simulink model "truck_fra_oven_konstant_hastighet"  (R2023b)
settings: Solver=VariableStepAuto  StartTime=0.0  StopTime=30  MaxStep=0.01  RelTol=1e-3
values from neighbouring files (symbols this model uses):
  k_1 = -0.1    [truck_fra_oven_konstant_hastighet_script.m]
  k_2 = 2    [truck_fra_oven_konstant_hastighet_script.m]
  y_r = 2    [truck_fra_oven_konstant_hastighet_script.m]
settings Model: Creator=hansae  LastModifiedBy=fredr
settings SolverCC: AlgebraicLoopSolver=TrustRegion
settings SFSimCC: CustomCodeUndefinedFunction=UseInterfaceOnly

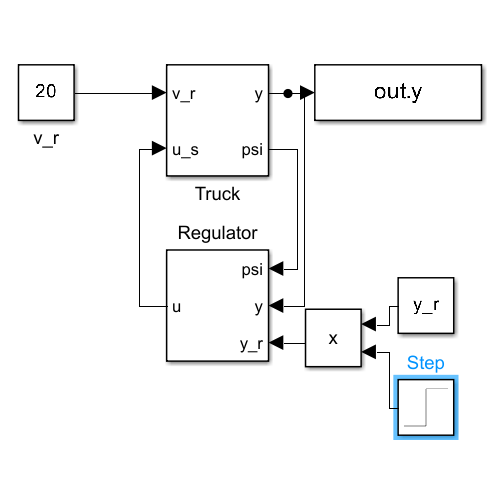
[thumbnail: Simulink's stored preview of the top-level diagram]
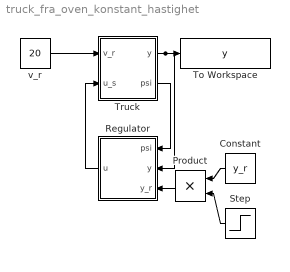
== system truck_fra_oven_konstant_hastighet ==
  Constant : Constant  Value=y_r
  Product : Product
  Regulator : Subsystem
  Step : Step  Time=10  Before=-1  SampleTime=0
  To Workspace : ToWorkspace  VariableName=y  SampleTime=-1
  Truck : Subsystem
  v_r : Constant  Value=20
  wires:
  v_r/1 -> Truck/1(v_r)
  Regulator/1(u) -> Truck/2(u_s)
  Truck/2(psi) -> Regulator/1(psi)
  Truck/1(y) -> To Workspace/1, Regulator/2(y)
  Product/1 -> Regulator/3(y_r)
  Constant/1 -> Product/1
  Step/1 -> Product/2

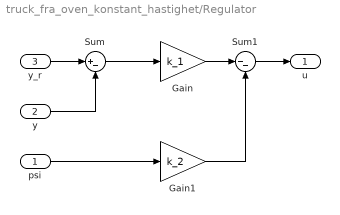
== system truck_fra_oven_konstant_hastighet/Regulator ==
  psi : Inport
  y : Inport  Port=2
  y_r : Inport  Port=3
  Gain : Gain  Gain=k_1
  Gain1 : Gain  Gain=k_2
  Sum : Sum  Inputs=|+-
  Sum1 : Sum  Inputs=|--
  u : Outport
  wires:
  y_r/1 -> Sum/1
  y/1 -> Sum/2
  Sum/1 -> Gain/1
  psi/1 -> Gain1/1
  Gain/1 -> Sum1/1
  Sum1/1 -> u/1
  Gain1/1 -> Sum1/2

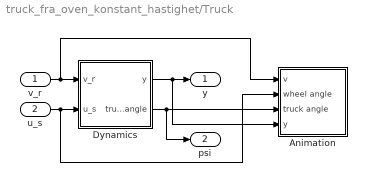
== system truck_fra_oven_konstant_hastighet/Truck ==
  v_r : Inport
  u_s : Inport  Port=2
  Animation : Subsystem
  Dynamics : Subsystem  ClipboardFcn=parameters_truck.m
  y : Outport
  psi : Outport  Port=2
  wires:
  Dynamics/1(y) -> Animation/4(y), y/1
  u_s/1 -> Animation/2(wheel angle), Dynamics/2(u_s)
  v_r/1 -> Animation/1(v), Dynamics/1(v_r)
  Dynamics/2(truck angle) -> psi/1, Animation/3(truck angle)

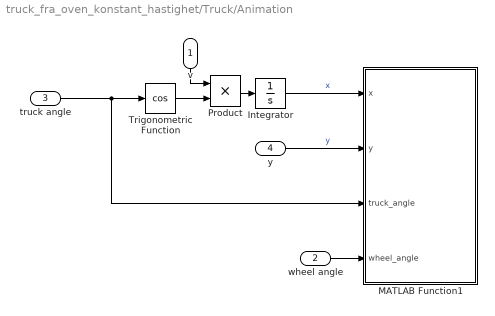
== system truck_fra_oven_konstant_hastighet/Truck/Animation ==
  v : Inport
  wheel angle : Inport  Port=2
  truck angle : Inport  Port=3
  y : Inport  Port=4
  Integrator : Integrator
  MATLAB Function1 : MATLAB Function  TreatAsAtomicUnit=on  SystemSampleTime=1/30
  Product : Product
  Trigonometric Function : Trigonometry  Operator=cos
  wires:
  Product/1 -> Integrator/1
  Trigonometric Function/1 -> Product/2
  v/1 -> Product/1
  y/1 -> MATLAB Function1/2(y)  "y"
  Integrator/1 -> MATLAB Function1/1(x)  "x"
  truck angle/1 -> MATLAB Function1/3(truck_angle), Trigonometric Function/1
  wheel angle/1 -> MATLAB Function1/4(wheel_angle)

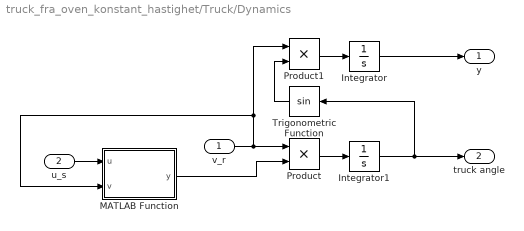
== system truck_fra_oven_konstant_hastighet/Truck/Dynamics ==
  v_r : Inport
  u_s : Inport  Port=2
  Integrator : Integrator  InitialCondition=-2
  Integrator1 : Integrator
  MATLAB Function : MATLAB Function  TreatAsAtomicUnit=on
  Product : Product
  Product1 : Product
  Trigonometric Function : Trigonometry
  y : Outport
  truck angle : Outport  Port=2
  wires:
  Integrator/1 -> y/1
  Integrator1/1 -> truck angle/1, Trigonometric Function/1
  Product/1 -> Integrator1/1
  v_r/1 -> MATLAB Function/2(v), Product1/1, Product/1
  Product1/1 -> Integrator/1
  Trigonometric Function/1 -> Product1/2
  u_s/1 -> MATLAB Function/1(u)
  MATLAB Function/1(y) -> Product/2

== matlab function truck_fra_oven_konstant_hastighet/Truck/Dynamics/MATLAB Function ==
  data: u input; y output; v input
function y = saturation(u,v)
    Pmax = 400000;
    epsilon = 0.1;
    
    sat = Pmax/sqrt(v^2+epsilon);
    y = max(min(u,sat),-sat);

== matlab function truck_fra_oven_konstant_hastighet/Truck/Animation/MATLAB Function1 ==
  settings: updateMethod=DISCRETE
  data: x input; y input; truck_angle input; wheel_angle input
function plot_truck(x,y,truck_angle,wheel_angle)
    % Parameters
    l = 8;
    persistent Truck;

    % Plotting Truck
    if isempty(Truck)
        Truck = initialize_plot();
    else
        update_truck_position(Truck,x,y,truck_angle,wheel_angle);
    end    

    drawnow;

    % Functions
    function Truck = initialize_plot()
        % Create figure
        figure('position',[100,100,1500,500]);
        clf; grid on; hold on; daspect([1,1,1]);
        xlim([-20, 50])
        ylim([-10, 10])
    
        % Road
        plot([-5000,5000],[-4,-4],'k','linewidth',3);
        plot([-5000,5000],[4,4],'k','linewidth',3);
        plot([-5000,5000],[0,0],'y','linewidth',3);

        % Truck
        Truck               = hgtransform('parent',gca);
        Left_front_wheel    = hgtransform('parent',Truck);
        Right_front_wheel   = hgtransform('parent',Truck);

        % Back wheels
        rectangle('Position',[l/6,-l/100,l/8,l/40],'parent',Truck,'edgecolor','k','linewidth',2,'FaceColor','w')
        rectangle('Position',[l/6,l-2*l/3-(l/40-l/100),l/8,l/40],'parent',Truck,'edgecolor','k','linewidth',2,'FaceColor','w')
        % Front wheel
        rectangle('Position',[2*l/3+l/20,-l/100,l/8,l/40],'parent',Right_front_wheel,'edgecolor','k','linewidth',2,'FaceColor','w')
        rectangle('Position',[2*l/3+l/20,l-2*l/3-(l/40-l/100),l/8,l/40],'parent',Left_front_wheel,'edgecolor','k','linewidth',2,'FaceColor','w')
        % Back
        rectangle('Position',[0,0,11*l/18,l-2*l/3],'parent',Truck,'edgecolor','k','linewidth',2,'FaceColor','w')
        % Front
        rectangle('Position',[2*l/3,0,l-2*l/3,l-2*l/3],'parent',Truck,'edgecolor','k','linewidth',2,'FaceColor','w')
        % Connection
        rectangle('Position',[11*l/18,3*l/8-l/3,2*l/3-11*l/18,l-3*l/4],'parent',Truck,'edgecolor','k','linewidth',2,'FaceColor','w')
        % Window
        rectangle('Position',[7*l/8,0,l/8,l-2*l/3],'parent',Truck,'edgecolor','k','linewidth',2,'FaceColor','w')
        
    end
    
    function update_truck_position(Truck,x,y,truck_angle,wheel_angle)
        if ishandle(Truck)
            set(Truck, 'Matrix', makehgtform('translate', [x, y, 0], 'zrotate', truck_angle, 'translate', [-l/6-l/16, -l/2+l/3, 0]));
            
            children = get(Truck, 'Children');
            set(children(8), 'Matrix', makehgtform('translate', -[-(2*l/3+l/20)-l/16, -(l-2*l/3-(l/40-l/100))-l/80, 0], 'zrotate', -wheel_angle, 'translate', [-(2*l/3+l/20)-l/16, -(l-2*l/3-(l/40-l/100))-l/80, 0]));
            set(children(7), 'Matrix', makehgtform('translate', -[-(2*l/3+l/20)-l/16, l/100-l/80, 0], 'zrotate', -wheel_angle, 'translate', [-(2*l/3+l/20)-l/16, l/100-l/80, 0]));
    
            xlim([-20, 50] + x)
            ylim([-10, 10] + y)
        end
    end
end
